simulink model "distMoment"  (R2023b)
settings: Solver=VariableStepAuto  StartTime=0.0  StopTime=10.0  RelTol=1e-3
settings Model: Creator=kristopherriordan  LastModifiedBy=kristopherriordan

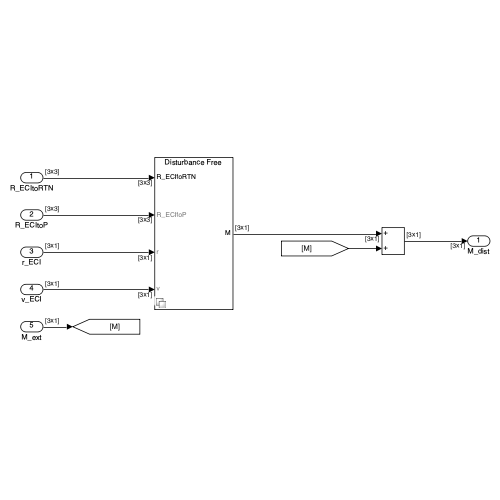
[thumbnail: Simulink's stored preview of the top-level diagram]
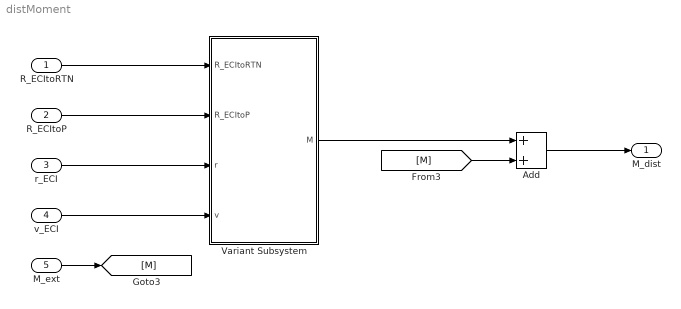
== system distMoment ==
  R_ECItoRTN : Inport
  R_ECItoP : Inport  Port=2
  r_ECI : Inport  Port=3
  v_ECI : Inport  Port=4
  M_ext : Inport  Port=5  PortDimensions=[3 1]
  Add : Sum
  Variant Subsystem : Subsystem  Variant=on
  M_dist : Outport
  wires:
  M_ext/1 -> [M]
  R_ECItoRTN/1 -> Variant Subsystem/1(R_ECItoRTN)
  r_ECI/1 -> Variant Subsystem/3(r)
  v_ECI/1 -> Variant Subsystem/4(v)
  Variant Subsystem/1(M) -> Add/1
  [M] -> Add/2
  R_ECItoP/1 -> Variant Subsystem/2(R_ECItoP)
  Add/1 -> M_dist/1

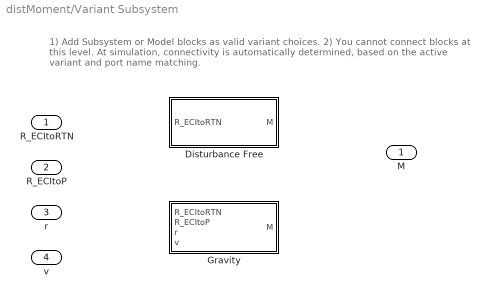
== system distMoment/Variant Subsystem ==
  note: 1) Add Subsystem or Model blocks as valid variant choices.
      | 2) You cannot connect blocks at this level. At simulation, connectivity is automatically
      | determined, based on the active variant and port name matching.
  R_ECItoRTN : Inport  PortDimensions=[3 3]
  R_ECItoP : Inport  Port=2  PortDimensions=[3 3]
  r : Inport  Port=3  PortDimensions=[3 1]
  v : Inport  Port=4  PortDimensions=[3 1]
  Disturbance Free : Subsystem  VariantControl="disturbance==\"none\""
  Gravity : Subsystem  VariantControl="disturbance==\"grav\""
  M : Outport

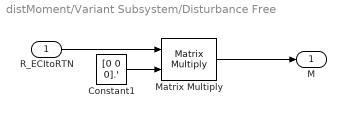
== system distMoment/Variant Subsystem/Disturbance Free ==
  R_ECItoRTN : Inport
  Constant1 : Constant  Value=[0 0 0].'  VectorParams1D=off
  Matrix Multiply : Product  Multiplication=Matrix(*)
  M : Outport
  wires:
  Matrix Multiply/1 -> M/1
  R_ECItoRTN/1 -> Matrix Multiply/1
  Constant1/1 -> Matrix Multiply/2

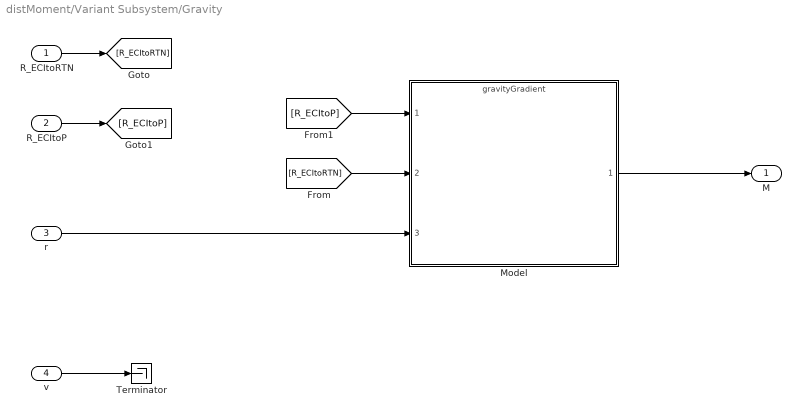
== system distMoment/Variant Subsystem/Gravity ==
  R_ECItoRTN : Inport
  R_ECItoP : Inport  Port=2
  r : Inport  Port=3
  v : Inport  Port=4
  Model : ModelReference  ModelNameDialog=gravityGradient.slx  SimulationMode=Normal  ModelReferenceVersion=1.2
  Terminator : Terminator
  M : Outport
  wires:
  R_ECItoRTN/1 -> [R_ECItoRTN]
  R_ECItoP/1 -> [R_ECItoP]
  [R_ECItoP] -> Model/1
  [R_ECItoRTN] -> Model/2
  r/1 -> Model/3
  Model/1 -> M/1
  v/1 -> Terminator/1
